simulink model "finalcode"  (R2020a)
settings: Solver=FixedStepDiscrete  StartTime=0.0  StopTime=1  FixedStep=0.0005  RelTol=1e-3  EnableMultiTasking=on
undefined symbols (not defined in the file): acc_calmax1, acc_calmax2, acc_calmin1, acc_calmin2, akemancanshu, angle_middle, bre, bre_calmax, bre_calmin, chasuniujvvvv_hou, chasuniujvvvv_qian, chasuuuu, ecucoder_acal, I_AN01_5K1, I_AN03_5V, I_AN04_5V, kd, kddd, ki, kiii, kp, kppp, leftmax, O_SW06_HS1A, P11111, P22222, PIDmodel, PPPP, rightmax, slip, slip_big, slip_little, slipmodel, T_add, T_del, tiaoshi, TTTTTyouren, vvvv, zhiling
libraries: ec5744lib x305, canmsglib x97, simulink x23
(part 10 of 11)

== matlab function finalcode/Subsystem/run/analog_input/无人意图转译/无人/Subsystem1/进esc控制策略/integral ==
  data: u input; output output; vd input
function output = fcn(u,vd)
    % 赛车PID控制器参数
    kp = 1;
    ki = 0.1;
    kd = 0.1;
    
    % 状态变量
    persistent pre_integral previous_error i
    
    % 初始化状态变量
    if isempty(pre_integral)
        pre_integral = 0;
        previous_error = 0;
        i=0;
    end
        if i>50
            i=0;
        end
    % PID控制器计算
    error = u;
    integral = pre_integral + error*0.02;
    derivative = (error - previous_error)/0.02;
%     integral =0;
    if abs(error)<0.1
        ki=0;
    end
    output = kp * error + ki * integral + kd * derivative;
    
   if vd==0
       output=0;
   end
    % 保存上一个误差用于下次计算
    previous_error = error;
    pre_integral =integral ;
    i=i+1
end

== matlab function finalcode/Subsystem/run/analog_input/无人意图转译/无人/Subsystem1/进esc控制策略/MATLAB Function1 ==
  data: output input; u input; y output; v input; vd input
function y = fcn(output, u,v,vd)
persistent vv
if isempty(vv)
    vv=0;
end
vv=output;
if v-vd>0.1*v
    y=vv;
else
    y=u;
end

== matlab function finalcode/Subsystem/run/analog_input/有人/功率限制jiandan/MATLAB Function ==
  data: u1 input; y output; u2 input; u3 input; u4 input
function y = fcn(u1,u2,u3,u4)
sum=(u1+u2+u3+u4)*594.06/1000/9550;
if sum>75
   a=75/sum;
else
    a=1;
end
y = a;

== matlab function finalcode/Subsystem/run/analog_input/有人/扭矩分配jiandan/MATLAB Function1 ==
  data: fengzhiniuju input; ax input; ay input
function fcn(fengzhiniuju,ax, ay)

end

== matlab function finalcode/Subsystem/run/analog_input/有人/扭矩分配jiandan/MATLAB Function3 ==
  data: M_qian input; M_hou input; youhou output; M input; youqian output; zuohou output; zuoqian output; you input; zuo input
function [youhou,youqian,zuohou,zuoqian] = fcn(M_qian,M_hou,M,you,zuo)
% U=4*u;
r=0.2032;%轮半径
B1=1.18;%左右轮距
B2=1.16;
youqian=you*(M*r/(2*B2)+M_qian);
zuoqian=zuo*(-M*r/(2*B1)+M_qian);
youhou=you*(M*r/(2*B2)+M_hou);
zuohou=zuo*(-M*r/(2*B1)+M_hou);
end

== matlab function finalcode/Subsystem/run/analog_input/无人意图转译/无人/Subsystem1/进esc控制策略/MATLAB Function2 ==
  data: u input; y output
function y = fcn(u)
persistent pre_Torque i
   
    % 初始化状态变量
    if isempty(pre_Torque)
          pre_Torque = 0;
          
        i=0;
    end
    if pre_Torque>u
   Torque= pre_Torque-100;
    else 
     Torque= pre_Torque;   
    end
  
    if  Torque<u
       Torque=u;
    end
    
    pre_Torque = Torque;

    i=i+1;
y = Torque;

== matlab function finalcode/Subsystem/Tx/TX控制器/控制器发送/184左前1/MATLAB Function ==
  data: u input; y output; zhidongesc input; zhidongebs input; huanting input
function y = fcn(u,zhidongesc,zhidongebs,huanting)
 y = u*594.06;
if zhidongesc>1800&&zhidongebs==2
    y = u*594.06;
end
if zhidongesc<1500&&zhidongebs==2
    y=0;
end
if huanting==0
    y=0;
end

== matlab function finalcode/Subsystem/Tx/TX控制器/控制器发送/184左前1/MATLAB Function1 ==
  data: v input; T output; a input
function T = fcn(v,a)
% if a>5
%     y = u;
% elseif a>3&&a<5
%     y=1200;
% else
%     y=800;
% end

if v<6000*1.88e-3
    T=2100;
elseif v>11000*1.88e-3
    T=800;
else
    T=1100;
end

== matlab function finalcode/Subsystem/Tx/TX控制器/控制器发送/184左前1/MATLAB Function3 ==
  data: v input; y output; angle input; vz input; model input
function y = fcn(v, angle, vz,model)
if(angle>3||angle<-3)&&model==3%4650000,4870000,4741002
    y=vz*594.06;
else
    y = v;
end

== matlab function finalcode/Subsystem/Tx/TX控制器/控制器发送/184左前1/MATLAB Function4 ==
  data: NT output; pos input; TargetVelocity input; T output; neg input; wheel_v input; v output
function [NT,T,v]= fcn(pos,TargetVelocity, neg,wheel_v)
persistent new_Torque i
    % 初始化状态变量
    if isempty(new_Torque)
          new_Torque = 0;  
          i=0;
    end
    if neg<0 && i==0;  %反扭
        v=0;
        i=1;
        new_Torque = pos;
    elseif i==1 && neg<0 && new_Torque>neg && new_Torque>=0;
        v=0;
        new_Torque=new_Torque-200;
    elseif i==1 && neg<0 && new_Torque>neg && new_Torque<0;
        v=0;
        new_Torque=new_Torque-50;
    elseif i==1 && neg<0 && new_Torque<=neg;
        v=0;
        new_Torque=neg;
    else %正扭矩情况
        v=TargetVelocity;
        i=0;
    end
    
    if neg<0 && new_Torque>=0
        T=new_Torque;
        NT=0;
    elseif neg<0 && new_Torque<0
        T=0;
        NT=new_Torque;
    else %正扭矩
        T=pos;
        NT=0;
    end
    
    if wheel_v<1
  v=TargetVelocity;
end

== matlab function finalcode/Subsystem/Tx/TX控制器/控制器发送/184左前1/MATLAB Function7 ==
  data: T input; y output; wurenyouya input; youya input; enable input; enable_1 input
function y = fcn(T, wurenyouya,youya, enable, enable_1)
 y = 0;
if wurenyouya>10||youya>500
    y = T;
else
    y=0;
end
if enable==0
    y=0;
end

== matlab function finalcode/Subsystem/Tx/TX控制器/控制器发送/184左前1/复位 ==
  data: enable input; enable_1 input; T input; TargetVelocity output; AMK_TorqueLimitPositive output; enable output; errorreset output; blnverteron output; CAN_dbcon output; v input
function [TargetVelocity,AMK_TorqueLimitPositive,enable,errorreset,blnverteron,CAN_dbcon]= fcn(enable,enable_1,T,v)
if (enable_1==0)
    TargetVelocity=0;
    enable=0;
    errorreset=1;
    blnverteron=0;
    CAN_dbcon=0;
    AMK_TorqueLimitPositive=0;
elseif (enable==0 && enable_1==1)
    TargetVelocity=0;
    enable=1;
    errorreset=0;
    blnverteron=1;
    CAN_dbcon=1;
    AMK_TorqueLimitPositive=0;
elseif (enable==1 && enable_1==1)
    TargetVelocity=v;
    enable=1;
    errorreset=0;
    blnverteron=1;
    CAN_dbcon=1;
    AMK_TorqueLimitPositive=T;
else
    TargetVelocity=0;
    enable=0;
    errorreset=1;
    blnverteron=0;
    CAN_dbcon=0;
    AMK_TorqueLimitPositive=0;
end

end

== matlab function finalcode/Subsystem/Tx/TX控制器/速度/185右前/MATLAB Function4 ==
  data: u input; y output; zhidongesc input; zhidongebs input; huanting input
function y = fcn(u,zhidongesc,zhidongebs,huanting)
 y = u*594.06;
if zhidongesc>1800&&zhidongebs==2
    y = u*594.06;
end
if zhidongesc<1500&&zhidongebs==2
    y=0;
end
if huanting~=0
    y=0;
end

== matlab function finalcode/Subsystem/Tx/TX控制器/控制器发送/184左前1/无人模式速度判断 ==
  data: u input; y output; zhidongesc input; zhidongebs input; huanting input
function y = fcn(u,zhidongesc,zhidongebs,huanting)
 y = u*594.06;
if zhidongesc>1800&&zhidongebs==2
    y = u*594.06;
end
if zhidongesc<1500&&zhidongebs==2
    y=0;
end
if huanting~=0
    y=0;
end

== matlab function finalcode/Subsystem/Tx/TX控制器/控制器发送/184左前1/有人无人扭矩转换 ==
  data: angle input; baziniujv input; v input; youren input; T output; model input
function T = fcn(angle, baziniujv, v,youren, model)
% if a>5
%     y = u;
% elseif a>3&&a<5
%     y=1200;
% else
%     y=800;
% end

if model==0||model==9||model==10   %有人模式，调试模式
    T=youren;
elseif model==3||abs(angle)>3  %wurenbazi
        if baziniujv==0
            T_bazi=2100;
        else
            T_bazi=baziniujv;
        end
        
    if v<10000*1.88e-3
        T=T_bazi;
    elseif v>11000*1.88e-3
        T=800;
    else
        T=1100;
   end
else                    %无人模式
   if v<6000*1.88e-3
     T=2100;
    elseif v>11000*1.88e-3
        T=800;
    else
        T=1100;
   end
end

== matlab function finalcode/Subsystem/Tx/TX控制器/控制器发送/184左前1/有人无人速度转换 ==
  data: v input; y output; angle input; vz input; model input; zhidong input; T input; vk input; v_youren input
function y = fcn(v, angle, vz,model, zhidong, T, vk, v_youren)
if model==0||model==9||model==10  %有人模式/无人检查（电气）
    if zhidong==0
       y=v_youren;
    else 
        y=0;
    end
else                    %无人模式
    if model==3 %4650000,4870000,4741002 大角度且八字
        y=vz*594.06;
    elseif T >10
        y=0;
        if vk<1
            y=v*594.06;
        end
    else
        y = v;  
    end    
end

== matlab function finalcode/Subsystem/Tx/TX控制器/控制器发送/184左前1/能量回收功率限制/MATLAB Function ==
  data: youya input; T output; model input; status input; wurenyouya input; Negativ_T input
function T = fcn(youya, model, status, wurenyouya, Negativ_T)
    if model == 0||model==10  %有人模式
        if youya>500
            T = (youya-500)*Negativ_T/4000;%最大反扭1000
            if youya>4500
                T = Negativ_T;
            end
        else
            T = 0;
        end
        
    elseif model~=0&&model~=9&&model~=2  %无人模式
        if wurenyouya>10
            T = -wurenyouya
        elseif status==5||status==7
                T=-1500; 
           % T = -(wurenyouya-500)/4;%最大反扭1000
            %if wurenyouya>500&&status==5
             %   T = -1000;
            %end
        else
            T = 0;
        end
    else
        T = 0;
end

== matlab function finalcode/Subsystem/Tx/TX控制器/控制器发送/184左前1/能量回收功率限制/MATLAB Function1 ==
  data: er_T input; T output; Iq input; L_Iq input; L_er_T input
function T = fcn(er_T, Iq, L_Iq,L_er_T)
if er_T<0
    if abs(Iq)>abs(L_Iq)
        T = -abs(L_er_T);

    else
        T = -abs(er_T);
    end
else
    T=0;
end

== matlab function finalcode/Subsystem/Tx/TX控制器/控制器发送/185右前1/MATLAB Function ==
  data: u input; y output; zhidongesc input; zhidongebs input
function y = fcn(u,zhidongesc,zhidongebs)
 y = u*594.06;
if zhidongesc>1800&&zhidongebs==2
    y = u*594.06;
end
if zhidongesc<1500&&zhidongebs==2
    y=0;
end

== matlab function finalcode/Subsystem/Tx/TX控制器/控制器发送/185右前1/MATLAB Function1 ==
  data: v input; T output; a input
function T = fcn(v,a)
% if a>5
%     y = u;
% elseif a>3&&a<5
%     y=1200;
% else
%     y=800;
% end

if v<6000*1.88e-3
    T=2100;
elseif v>11000*1.88e-3
    T=800;
else
    T=1100;
end

== matlab function finalcode/Subsystem/Tx/TX控制器/控制器发送/185右前1/MATLAB Function2 ==
  data: enable input; enable_1 input; T input; TargetVelocity output; AMK_TorqueLimitPositive output; enable output; errorreset output; blnverteron output; CAN_dbcon output; v input
function [TargetVelocity,AMK_TorqueLimitPositive,enable,errorreset,blnverteron,CAN_dbcon]= fcn(enable,enable_1,T,v)
if (enable_1==0)
    TargetVelocity=0;
    enable=0;
    errorreset=1;
    blnverteron=0;
    CAN_dbcon=0;
    AMK_TorqueLimitPositive=0;
elseif (enable==0 && enable_1==1)
    TargetVelocity=0;
    enable=1;
    errorreset=0;
    blnverteron=1;
    CAN_dbcon=1;
    AMK_TorqueLimitPositive=0;
elseif (enable==1 && enable_1==1)
    TargetVelocity=v;
    enable=1;
    errorreset=0;
    blnverteron=1;
    CAN_dbcon=1;
    AMK_TorqueLimitPositive=T;
else
    TargetVelocity=0;
    enable=0;
    errorreset=1;
    blnverteron=0;
    CAN_dbcon=0;
    AMK_TorqueLimitPositive=0;
end

end

== matlab function finalcode/Subsystem/Tx/TX控制器/速度/185右前/MATLAB Function5 ==
  data: v input; y output; angle input; vz input; model input
function y = fcn(v, angle, vz,model)
if(angle>3||angle<-3)&&model==3%4650000,4870000,4741002
    y=vz*594.06;
else
    y = v;
end

== matlab function finalcode/Subsystem/Tx/TX控制器/控制器发送/185右前1/MATLAB Function3 ==
  data: v input; y output; angle input; vz input; model input
function y = fcn(v, angle, vz,model)
if (angle>3||angle<-3)&&model==3%4650000,4870000,4741002
    y=vz*594.06;
else
    y = v;
end

== matlab function finalcode/Subsystem/Tx/TX控制器/控制器发送/185右前1/MATLAB Function4 ==
  data: u input; y output; zhidongesc input; zhidongebs input; huanting input
function y = fcn(u,zhidongesc,zhidongebs,huanting)
 y = u*594.06;
if zhidongesc>1800&&zhidongebs==2
    y = u*594.06;
end
if zhidongesc<1500&&zhidongebs==2
    y=0;
end
if huanting~=0
    y=0;
end

== matlab function finalcode/Subsystem/Tx/TX控制器/控制器发送/185右前1/vvv ==
  data: v input; y output; angle input; vz input; model input; zhidong input; T input; vk input; v_youren input
function y = fcn(v, angle, vz,model, zhidong, T, vk, v_youren)
if model==0||model==9||model==10  %有人模式/无人检查（电气）
    if zhidong==0
       y=v_youren;
    else 
        y=0;
    end
else                    %无人模式
    if model==3 %4650000,4870000,4741002 大角度和八字状态
        y=vz*594.06;
    elseif T >10
        y=0;
        if vk<1
            y=v*594.06;
        end
    else
        y = v;
    end   
end

== matlab function finalcode/Subsystem/Tx/TX控制器/控制器发送/185右前1/MATLAB Function6 ==
  data: angle input; baziniujv input; v input; youren input; T output; model input
function T = fcn(angle, baziniujv, v,youren, model)
% if a>5
%     y = u;
% elseif a>3&&a<5
%     y=1200;
% else
%     y=800;
% end

if model==0||model==9||model==10   %有人模式，调试模式
    T=youren;
elseif model==3||abs(angle)>3  %wurenbazi
        if baziniujv==0
            T_bazi=2100;
        else
            T_bazi=baziniujv;
        end
        
    if v<10000*1.88e-3
        T=T_bazi;
    elseif v>11000*1.88e-3
        T=800;
    else
        T=1100;
   end
else                    %无人模式
   if v<6000*1.88e-3
     T=2100;
    elseif v>11000*1.88e-3
        T=800;
    else
        T=1100;
   end
end

== matlab function finalcode/Subsystem/Tx/TX控制器/控制器发送/185右前1/MATLAB Function7 ==
  data: T input; y output; wurenyouya input; youya input; enable input; enable_1 input
function y = fcn(T, wurenyouya,youya, enable, enable_1)
 y = 0;
if wurenyouya>10||youya>500
    y = T;
else
    y=0;
end
if enable==0
    y=0;
end

== matlab function finalcode/Subsystem/Tx/TX控制器/控制器发送/185右前1/MATLAB Function8 ==
  data: pos input; TargetVelocity input; NT output; T output; neg input; wheel_v input; v output
function [NT,T,v]= fcn(pos,TargetVelocity, neg,wheel_v)
persistent new_Torque i
    % 初始化状态变量
    if isempty(new_Torque)
          new_Torque = 0;  
          i=0;
    end
    if neg<0 && i==0;  %反扭
        v=0;
        i=1;
        new_Torque = pos;
    elseif i==1 && neg<0 && new_Torque>neg && new_Torque>=0;
        v=0;
        new_Torque=new_Torque-200;
    elseif i==1 && neg<0 && new_Torque>neg && new_Torque<0;
        v=0;
        new_Torque=new_Torque-50;
    elseif i==1 && neg<0 && new_Torque<=neg;
        v=0;
        new_Torque=neg;
    else %正扭矩情况
        v=TargetVelocity;
        i=0;
    end
    
    if neg<0 && new_Torque>=0
        T=new_Torque;
        NT=0;
    elseif neg<0 && new_Torque<0
        T=0;
        NT=new_Torque;
    else %正扭矩
        T=pos;
        NT=0;
    end
    
    if wheel_v<1
  v=TargetVelocity;
end

== matlab function finalcode/Subsystem/Tx/TX控制器/控制器发送/185右前1/能量回收功率限制/MATLAB Function ==
  data: youya input; T output; model input; status input; wurenyouya input; Negativ_T input
function T = fcn(youya, model, status, wurenyouya, Negativ_T)
    if model == 0||model==10  %有人模式
        if youya>500
            T = (youya-500)*Negativ_T/4000;%最大反扭1000
            if youya>4500
                T = Negativ_T;
            end
        else
            T = 0;
        end
        
    elseif model~=0&&model~=9&&model~=2  %无人模式
        if wurenyouya>10
            T = -wurenyouya
        elseif status==5||status==7
                T=-1500;
           % T = -(wurenyouya-500)/4;%最大反扭1000
            %if wurenyouya>500&&status==5
             %   T = -1000;
            %end
        else
            T = 0;
        end
    else
        T = 0;
end

== matlab function finalcode/Subsystem/Tx/TX控制器/控制器发送/185右前1/能量回收功率限制/MATLAB Function1 ==
  data: er_T input; T output; Iq input; L_Iq input; L_er_T input
function T = fcn(er_T, Iq, L_Iq,L_er_T)
if er_T<0
    if abs(Iq)>abs(L_Iq)
        T = -abs(L_er_T);

    else
        T = -abs(er_T);
    end
else
    T=0;
end

== matlab function finalcode/Subsystem/Tx/TX控制器/控制器发送/188右后1/MATLAB Function ==
  data: u input; y output; zhidongesc input; zhidongebs input
function y = fcn(u,zhidongesc,zhidongebs)
 y = u*594.06;
if zhidongesc>1800&&zhidongebs==2
    y = u*594.06;
end
if zhidongesc<1500&&zhidongebs==2
    y=0;
end

== matlab function finalcode/Subsystem/Tx/TX控制器/控制器发送/188右后1/MATLAB Function1 ==
  data: v input; T output; a input
function T = fcn(v,a)
% if a>5
%     y = u;
% elseif a>3&&a<5
%     y=1200;
% else
%     y=800;
% end

if v<6000*1.88e-3
    T=2100;
elseif v>11000*1.88e-3
    T=800;
else
    T=1100;
end

== matlab function finalcode/Subsystem/Tx/TX控制器/速度/185右前/MATLAB Function6 ==
  data: v input; T output; a input
function T = fcn(v,a)
% if a>5
%     y = u;
% elseif a>3&&a<5
%     y=1200;
% else
%     y=800;
% end

if v<6000*1.88e-3
    T=2100;
elseif v>11000*1.88e-3
    T=800;
else
    T=1100;
end

== matlab function finalcode/Subsystem/Tx/TX控制器/控制器发送/188右后1/MATLAB Function2 ==
  data: enable input; enable_1 input; T input; TargetVelocity output; AMK_TorqueLimitPositive output; enable output; errorreset output; blnverteron output; CAN_dbcon output; v input
function [TargetVelocity,AMK_TorqueLimitPositive,enable,errorreset,blnverteron,CAN_dbcon]= fcn(enable,enable_1,T,v)
if (enable_1==0)
    TargetVelocity=0;
    enable=0;
    errorreset=1;
    blnverteron=0;
    CAN_dbcon=0;
    AMK_TorqueLimitPositive=0;
elseif (enable==0 && enable_1==1)
    TargetVelocity=0;
    enable=1;
    errorreset=0;
    blnverteron=1;
    CAN_dbcon=1;
    AMK_TorqueLimitPositive=0;
elseif (enable==1 && enable_1==1)
    TargetVelocity=v;
    enable=1;
    errorreset=0;
    blnverteron=1;
    CAN_dbcon=1;
    AMK_TorqueLimitPositive=T;
else
    TargetVelocity=0;
    enable=0;
    errorreset=1;
    blnverteron=0;
    CAN_dbcon=0;
    AMK_TorqueLimitPositive=0;
end

end

== matlab function finalcode/Subsystem/Tx/TX控制器/控制器发送/188右后1/MATLAB Function3 ==
  data: v input; y output; angle input; vz input; model input
function y = fcn(v, angle,vz,model)
if (angle>3||angle<-3)&&model==3%4650000,4870000,4741002
    y=vz*594.06;
else
    y = v;
end

== matlab function finalcode/Subsystem/Tx/TX控制器/控制器发送/188右后1/MATLAB Function4 ==
  data: u input; y output; zhidongesc input; zhidongebs input; huanting input
function y = fcn(u,zhidongesc,zhidongebs,huanting)
 y = u*594.06;
if zhidongesc>1800&&zhidongebs==2
    y = u*594.06;
end
if zhidongesc<1500&&zhidongebs==2
    y=0;
end
if huanting~=0
    y=0;
end

== matlab function finalcode/Subsystem/Tx/TX控制器/控制器发送/188右后1/MATLAB Function5 ==
  data: v input; y output; angle input; vz input; model input; zhidong input; T input; vk input; v_youren input
function y = fcn(v, angle, vz,model, zhidong, T, vk, v_youren)
if model==0||model==9||model==10  %有人模式/无人检查（电气）
    if zhidong==0
       y=v_youren;
    else 
        y=0;
    end
else                    %无人模式
    if model==3 %4650000,4870000,4741002 大角度和八字状态
        y=vz*594.06;
    elseif T >10
        y=0;
        if vk<1
            y=v*594.06;
        end
    else
        y = v;
    end    
end

== matlab function finalcode/Subsystem/Tx/TX控制器/控制器发送/188右后1/MATLAB Function6 ==
  data: T input; y output; wurenyouya input; youya input; enable input; enable_1 input
function y = fcn(T, wurenyouya,youya, enable, enable_1)
 y = 0;
if wurenyouya>10||youya>500
    y = T;
else
    y=0;
end
if enable==0
    y=0;
end

== matlab function finalcode/Subsystem/Tx/TX控制器/控制器发送/188右后1/MATLAB Function7 ==
  data: angle input; baziniujv input; v input; youren input; T output; model input
function T = fcn(angle, baziniujv, v,youren, model)
% if a>5
%     y = u;
% elseif a>3&&a<5
%     y=1200;
% else
%     y=800;
% end

if model==0||model==9||model==10   %有人模式，调试模式
    T=youren;
elseif model==3||abs(angle)>3  %wurenbazi
        if baziniujv==0
            T_bazi=2100;
        else
            T_bazi=baziniujv;
        end
        
    if v<10000*1.88e-3
        T=T_bazi;
    elseif v>11000*1.88e-3
        T=800;
    else
        T=1100;
   end
else                    %无人模式
   if v<6000*1.88e-3
     T=2100;
    elseif v>11000*1.88e-3
        T=800;
    else
        T=1100;
   end
end

== matlab function finalcode/Subsystem/Tx/TX控制器/控制器发送/188右后1/MATLAB Function9 ==
  data: pos input; TargetVelocity input; NT output; T output; neg input; wheel_v input; v output
function [NT,T,v]= fcn(pos,TargetVelocity, neg,wheel_v)
persistent new_Torque i
    % 初始化状态变量
    if isempty(new_Torque)
          new_Torque = 0;  
          i=0;
    end
    if neg<0 && i==0;  %反扭
        v=0;
        i=1;
        new_Torque = pos;
    elseif i==1 && neg<0 && new_Torque>neg && new_Torque>=0;
        v=0;
        new_Torque=new_Torque-200;
    elseif i==1 && neg<0 && new_Torque>neg && new_Torque<0;
        v=0;
        new_Torque=new_Torque-50;
    elseif i==1 && neg<0 && new_Torque<=neg;
        v=0;
        new_Torque=neg;
    else %正扭矩情况
        v=TargetVelocity;
        i=0;
    end
    
    if neg<0 && new_Torque>=0
        T=new_Torque;
        NT=0;
    elseif neg<0 && new_Torque<0
        T=0;
        NT=new_Torque;
    else %正扭矩
        T=pos;
        NT=0;
    end
    
    if wheel_v<1
  v=TargetVelocity;
end

== matlab function finalcode/Subsystem/Tx/Toworkstation/toworkstation/toworkstation/MATLAB Function ==
  data: T input; y output; NT input
function y = fcn(T, NT)

y = T;
if NT<-10
    y=NT;
end

== matlab function finalcode/Subsystem/Tx/TX控制器/控制器发送/188右后1/能量回收功率限制/MATLAB Function ==
  data: youya input; T output; model input; status input; wurenyouya input; Negativ_T input
function T = fcn(youya, model, status, wurenyouya, Negativ_T)
    if model == 0||model==10  %有人模式
        if youya>500
            T = (youya-500)*Negativ_T/4000;%最大反扭1000
            if youya>4500
                T = Negativ_T;
            end
        else
            T = 0;
        end
        
    elseif model~=0&&model~=9&&model~=2  %无人模式
        if wurenyouya>10
            T = -wurenyouya
        elseif status==5||status==7
                T=-1500;
           % T = -(wurenyouya-500)/4;%最大反扭1000
            %if wurenyouya>500&&status==5
             %   T = -1000;
            %end
        else
            T = 0;
        end
    else
        T = 0;
end

== matlab function finalcode/Subsystem/Tx/TX控制器/控制器发送/188右后1/能量回收功率限制/MATLAB Function1 ==
  data: er_T input; T output; Iq input; L_Iq input; L_er_T input
function T = fcn(er_T, Iq, L_Iq,L_er_T)
if er_T<0
    if abs(Iq)>abs(L_Iq)
        T = -abs(L_er_T);

    else
        T = -abs(er_T);
    end
else
    T=0;
end

== matlab function finalcode/Subsystem/Tx/TX控制器/控制器发送/189左后1/MATLAB Function ==
  data: u input; y output; zhidongesc input; zhidongebs input
function y = fcn(u,zhidongesc,zhidongebs)
 y = u*594.06;
if zhidongesc>1800&&zhidongebs==2
    y = u*594.06;
end
if zhidongesc<1500&&zhidongebs==2
    y=0;
end

== matlab function finalcode/Subsystem/Tx/TX控制器/控制器发送/189左后1/MATLAB Function1 ==
  data: v input; T output; a input
function T = fcn(v,a)
% if a>5
%     y = u;
% elseif a>3&&a<5
%     y=1200;
% else
%     y=800;
% end

if v<6000*1.88e-3
    T=2100;
elseif v>11000*1.88e-3
    T=800;
else
    T=1100;
end

== matlab function finalcode/Subsystem/Tx/TX控制器/控制器发送/189左后1/MATLAB Function2 ==
  data: enable input; enable_1 input; T input; TargetVelocity output; AMK_TorqueLimitPositive output; enable output; errorreset output; blnverteron output; CAN_dbcon output; v input
function [TargetVelocity,AMK_TorqueLimitPositive,enable,errorreset,blnverteron,CAN_dbcon]= fcn(enable,enable_1,T,v)
if (enable_1==0)
    TargetVelocity=0;
    enable=0;
    errorreset=1;
    blnverteron=0;
    CAN_dbcon=0;
    AMK_TorqueLimitPositive=0;
elseif (enable==0 && enable_1==1)
    TargetVelocity=0;
    enable=1;
    errorreset=0;
    blnverteron=1;
    CAN_dbcon=1;
    AMK_TorqueLimitPositive=0;
elseif (enable==1 && enable_1==1)
    TargetVelocity=v;
    enable=1;
    errorreset=0;
    blnverteron=1;
    CAN_dbcon=1;
    AMK_TorqueLimitPositive=T;
else
    TargetVelocity=0;
    enable=0;
    errorreset=1;
    blnverteron=0;
    CAN_dbcon=0;
    AMK_TorqueLimitPositive=0;
end

end

== matlab function finalcode/Subsystem/Tx/TX控制器/控制器发送/189左后1/MATLAB Function3 ==
  data: v input; y output; angle input; vz input; model input
function y = fcn(v, angle, vz,model)
if (angle>3||angle<-3)&&model==3%4650000,4870000,4741002
    y=vz*594.06;
else
    y = v;
end

== matlab function finalcode/Subsystem/Tx/TX控制器/控制器发送/189左后1/MATLAB Function4 ==
  data: u input; y output; zhidongesc input; zhidongebs input; huanting input
function y = fcn(u,zhidongesc,zhidongebs,huanting)
 y = u*594.06;
if zhidongesc>1800&&zhidongebs==2
    y = u*594.06;
end
if zhidongesc<1500&&zhidongebs==2
    y=0;
end
if huanting~=0
    y=0;
end

== matlab function finalcode/Subsystem/Tx/Toworkstation/toworkstation/toworkstation/MATLAB Function1 ==
  data: T input; y output; NT input
function y = fcn(T, NT)

y = T;
if NT<-10
    y=NT;
end

== matlab function finalcode/Subsystem/Tx/TX控制器/控制器发送/189左后1/MATLAB Function5 ==
  data: v input; y output; angle input; vz input; model input; zhidong input; T input; vk input; v_youren input
function y = fcn(v, angle, vz,model, zhidong, T, vk, v_youren)
if model==0||model==9||model==10  %有人模式/无人检查（电气）
    if zhidong==0
       y=v_youren;
    else 
        y=0;
    end
else                    %无人模式
    if model==3 %4650000,4870000,4741002 大角度和八字状态
        y=vz*594.06;
    elseif T >10
        y=0;
        if vk<1
            y=v*594.06;
        end
    else
        y = v;   
    end     
end

== matlab function finalcode/Subsystem/Tx/TX控制器/控制器发送/189左后1/MATLAB Function6 ==
  data: angle input; baziniujv input; v input; youren input; T output; model input
function T = fcn(angle, baziniujv, v,youren, model)
% if a>5
%     y = u;
% elseif a>3&&a<5
%     y=1200;
% else
%     y=800;
% end

if model==0||model==9||model==10   %有人模式，调试模式
    T=youren;
elseif model==3||abs(angle)>3  %wurenbazi
        if baziniujv==0
            T_bazi=2100;
        else
            T_bazi=baziniujv;
        end
        
    if v<10000*1.88e-3
        T=T_bazi;
    elseif v>11000*1.88e-3
        T=800;
    else
        T=1100;
   end
else                    %无人模式
   if v<6000*1.88e-3
     T=2100;
    elseif v>11000*1.88e-3
        T=800;
    else
        T=1100;
   end
end

== matlab function finalcode/Subsystem/Tx/TX控制器/控制器发送/189左后1/MATLAB Function7 ==
  data: T input; y output; wurenyouya input; youya input; enable input; enable_1 input
function y = fcn(T, wurenyouya,youya, enable, enable_1)
 y = 0;
if wurenyouya>10||youya>500
    y = T;
else
    y=0;
end
if enable==0
    y=0;
end

== matlab function finalcode/Subsystem/Tx/TX控制器/控制器发送/189左后1/MATLAB Function9 ==
  data: pos input; TargetVelocity input; NT output; T output; neg input; v output; wheel_v input
function [NT,T,v]= fcn(pos,TargetVelocity, neg,wheel_v)
persistent new_Torque i
    % 初始化状态变量
    if isempty(new_Torque)
          new_Torque = 0;  
          i=0;
    end
    if neg<0 && i==0;  %反扭
        v=0;
        i=1;
        new_Torque = pos;
    elseif i==1 && neg<0 && new_Torque>neg && new_Torque>=0;
        v=0;
        new_Torque=new_Torque-200;
    elseif i==1 && neg<0 && new_Torque>neg && new_Torque<0;
        v=0;
        new_Torque=new_Torque-50;
    elseif i==1 && neg<0 && new_Torque<=neg;
        v=0;
        new_Torque=neg;
    else %正扭矩情况
        v=TargetVelocity;
        i=0;
    end
    
    if neg<0 && new_Torque>=0
        T=new_Torque;
        NT=0;
    elseif neg<0 && new_Torque<0
        T=0;
        NT=new_Torque;
    else %正扭矩
        T=pos;
        NT=0;
    end
    
    if wheel_v<1
  v=TargetVelocity;
end

== matlab function finalcode/Subsystem/Tx/TX控制器/控制器发送/189左后1/能量回收功率限制/MATLAB Function ==
  data: youya input; T output; model input; status input; wurenyouya input; Negativ_T input
function T = fcn(youya, model, status, wurenyouya, Negativ_T)
    if model == 0||model==10  %有人模式
        if youya>500
            T = (youya-500)*Negativ_T/4000;%最大反扭1000
            if youya>4500
                T = Negativ_T;
            end
        else
            T = 0;
        end
        
    elseif model~=0&&model~=9&&model~=2  %无人模式
        if wurenyouya>10
            T = -wurenyouya
        elseif status==5||status==7
                T=-1500;
           % T = -(wurenyouya-500)/4;%最大反扭1000
            %if wurenyouya>500&&status==5
             %   T = -1000;
            %end
        else
            T = 0;
        end
    else
        T = 0;
end

== matlab function finalcode/Subsystem/Tx/TX控制器/控制器发送/189左后1/能量回收功率限制/MATLAB Function1 ==
  data: er_T input; T output; Iq input; L_Iq input; L_er_T input
function T = fcn(er_T, Iq, L_Iq,L_er_T)
if er_T<0
    if abs(Iq)>abs(L_Iq)
        T = -abs(L_er_T);

    else
        T = -abs(er_T);
    end
else
    T=0;
end

== matlab function finalcode/Subsystem/Tx/Toworkstation/toworkstation/toworkstation/MATLAB Function2 ==
  data: T input; y output; NT input
function y = fcn(T, NT)

y = T;
if NT<-10
    y=NT;
end

== matlab function finalcode/Subsystem/Tx/Toworkstation/toworkstation/toworkstation/MATLAB Function3 ==
  data: T input; y output; NT input
function y = fcn(T, NT)

y = T;
if NT<-10
    y=NT;
end

== matlab function finalcode/Subsystem/Rx/工作站/Subsystem3/Subsystem/MATLAB Function5 ==
  data: steer input; u input; y output; CANOK_20 input
function y = fcn(steer, u, CANOK_20)

% 初始化位数计数
num_digits = 0; 
% 处理0的情况
if u == 0
    num_digits = 1;
else
    % 计算位数
    num = abs(u);
    while num > 0
        num = floor(num / 10);
        num_digits = num_digits + 1;
    end
end
    divisor = 10 ^ num_digits;
    decimal = u / divisor;
    
    if steer>=0
        y=decimal;
    else
        y=-decimal;
    end
 
%     if CANOK_20==0
%     y=0;
%     end
end

== matlab function finalcode/Subsystem/Rx/工作站/Subsystem3/Subsystem/MATLAB Function3 ==
  data: steer input; u input; y output; CANOK_20 input
function y = fcn(steer, u,CANOK_20)
        y=u/100;

== matlab function finalcode/无人TX/Toworkstation/MATLAB Function ==
  data: u input; y output
function y = fcn(u)
if u~=0&&u~=9&&u~=2
    y=1;
else
    y=0;
end

== matlab function finalcode/Subsystem/Tx/TX控制器/速度/184左前/MATLAB Function2 ==
  data: enable input; enable_1 input; T input; TargetVelocity output; AMK_TorqueLimitPositive output; enable output; errorreset output; blnverteron output; CAN_dbcon output; v input
function [TargetVelocity,AMK_TorqueLimitPositive,enable,errorreset,blnverteron,CAN_dbcon]= fcn(enable,enable_1,T,v)
if (enable_1==0)
    TargetVelocity=0;
    enable=0;
    errorreset=1;
    blnverteron=0;
    CAN_dbcon=0;
    AMK_TorqueLimitPositive=0;
elseif (enable==0 && enable_1==1)
    TargetVelocity=2000;
    enable=1;
    errorreset=0;
    blnverteron=1;
    CAN_dbcon=1;
    AMK_TorqueLimitPositive=0;
elseif (enable==1 && enable_1==1)
    TargetVelocity=2000;
    enable=1;
    errorreset=0;
    blnverteron=1;
    CAN_dbcon=1;
    AMK_TorqueLimitPositive=T;
else
    TargetVelocity=0;
    enable=0;
    errorreset=1;
    blnverteron=0;
    CAN_dbcon=0;
    AMK_TorqueLimitPositive=0;
end

end

== matlab function finalcode/无人TX/Toworkstation/toworkstation/toworkstation/MATLAB Function ==
  data: T input; y output; NT input
function y = fcn(T, NT)

y = T;
if NT<-10
    y=NT;
end

== matlab function finalcode/无人TX/Toworkstation/toworkstation/toworkstation/MATLAB Function1 ==
  data: T input; y output; NT input
function y = fcn(T, NT)

y = T;
if NT<-10
    y=NT;
end

== matlab function finalcode/无人TX/Toworkstation/toworkstation/toworkstation/MATLAB Function2 ==
  data: T input; y output; NT input
function y = fcn(T, NT)

y = T;
if NT<-10
    y=NT;
end

== matlab function finalcode/Subsystem/Rx/lcu——receive/Subsystem1/Subsystem/MATLAB Function ==
  data: m input; y1 output; y2 output; y3 output
function [y1,y2,y3] = fcn(m)
V=zeros(1,3);
a=2;i=3;
while i>0
    V(1,i)=mod(m,a);
    m=fix(m/2);
    i=i-1;
end  
y1 = V(1,3);
y2=V(1,2);
y3=V(1,1);
end

== matlab function finalcode/Subsystem/Rx/lcu——receive/Subsystem1/Subsystem/MATLAB Function1 ==
  data: u input; y output
function y = fcn(u)
if u==7
    y = 1;
else
    y=0;
end
end

== matlab function finalcode/无人TX/Toworkstation/toworkstation/toworkstation/MATLAB Function3 ==
  data: T input; y output; NT input
function y = fcn(T, NT)

y = T;
if NT<-10
    y=NT;
end

== matlab function finalcode/Subsystem/Rx/工作站/Subsystem3/Subsystem/MATLAB Function6 ==
  data: u input; y output; CANOK_20 input
function y = fcn(u, CANOK_20)


% 初始化位数计数
num_digits = 0; 
% 处理0的情况
if u == 0
    num_digits = 1;
else
    % 计算位数
    num = abs(u);
    while num > 0
        num = floor(num / 10);
        num_digits = num_digits + 1;
    end
end
    divisor = 10 ^ num_digits;
    decimal = u / divisor;
    if u>0
        y=decimal;
    else
        y=-decimal;
    end
    if CANOK_20==0
    y=0;
    end
end

== matlab function finalcode/Subsystem/Rx/工作站/Subsystem3/Subsystem/MATLAB Function7 ==
  data: u input; y output; CANOK_20 input
function y = fcn(u,CANOK_20)
if CANOK_20==0
    y=0;
else
    y=u;
end

== matlab function finalcode/Subsystem/Rx/工作站/Subsystem3/Subsystem/MATLAB Function8 ==
  data: u input; y output; CANOK_20 input
function y = fcn(u, CANOK_20)
    if u==0
        y=0;
    else
        y=u/100;
    end
    
    if CANOK_20==0
    y=0;
    end
end

== matlab function finalcode/Subsystem/run/analog_input/无人意图转译/无人/Subsystem1/进esc控制策略/MATLAB Function3 ==
  data: v input; y output; v_k input
function y = fcn( v, v_k)
persistent pre_Torque a
   
    % 初始化状态变量
    if isempty(pre_Torque)
          pre_Torque = 0; 
            a=0;
    end
if v_k>v
    a=v-v_k;
else
    a=0;
end

if a<-0.5
    y=a;
else
    y=0;
end

== matlab function finalcode/Subsystem/Tx/TX控制器/控制器发送/184左前1/能量回收功率限制/P功率 ==
  data: P input; P1 input; P2 input; model input; y output
function y = fcn(P, P1, P2, model)
y=P;
if model==4||model==5  %循迹模式
    y=P1;
elseif model==1
    y=P2;
end

== matlab function finalcode/Subsystem/Tx/TX控制器/控制器发送/185右前1/能量回收功率限制/MATLAB Function2 ==
  data: P input; P1 input; P2 input; model input; y output
function y = fcn(P, P1, P2, model)
y=P;
if model==4||model==5  %循迹模式
    y=P1;
elseif model==1
    y=P2;
end

== matlab function finalcode/Subsystem/Tx/TX控制器/控制器发送/189左后1/能量回收功率限制/MATLAB Function2 ==
  data: P input; P1 input; P2 input; model input; y output
function y = fcn(P, P1, P2, model)
y=P;
if model==4||model==5  %循迹模式
    y=P1;
elseif model==1
    y=P2;
end

== matlab function finalcode/Subsystem/Tx/TX控制器/控制器发送/188右后1/能量回收功率限制/MATLAB Function2 ==
  data: P input; P1 input; P2 input; model input; y output
function y = fcn(P, P1, P2, model)
y=P;
if model==4||model==5  %循迹模式
    y=P1;
elseif model==1
    y=P2;
end

== matlab function finalcode/Subsystem/Tx/MATLAB Function ==
  data: u input; y output
function y = fcn(u)
if u==8
    y=1;
else
    y=0;
end

== matlab function finalcode/Subsystem/Tx/TX控制器/控制器发送/184左前1/滑移率控制 ==
  data: model input; v_e input; v_w input; v input; slipp input; y output; slip_little input; slip_big input
function y = fcn(model, v_e, v_w, v, slipp, slip_little, slip_big)
    persistent i j
    if isempty(i)
        i=1;
        j=1;
    end
if model==0
    y=v_e;
else
    slip=(v-v_w)/v;
    y=v_e;

    if abs(v_e-v_w)>0.5
        if slip_little==0  %调试用
            slip1=0.8;
        else
            slip1=slip_little;
        end
        if slip_big==0
            slip2=1.25;
        else
            slip2=slip_big;
        end
        if slipp==0
            slippp=0.21;
        else
            slippp=slipp;
        end
    if slip>slippp&&v_w>3; %减速，加大轮速
        y=j*v;
        i=i+1;
        j=0.99^i;
        if j<slip1
            j=slip1;
        end
    elseif slip<-slippp&&v_w>2%加速，缓加速
        y=j*v;
        i=i+1;
        j=1.01^i;
        if j>slip2
            j=slip2;
        end
    else
        y=v_e;
        i=1;
    end
    
    else
        y=v_e;
    end
    
    if v_e==0;
        y=0;
    end
end

== matlab function finalcode/Subsystem/run/analog_input/无人意图转译/无人/Subsystem1/MATLAB Function1 ==
  data: v input; model input; a1 input; a2 input; a3 input; a4 input; v1 input; v2 input; v3 input; v4 input; y1 output; y2 output; y3 output; y4 output
function [y1,y2,y3,y4] = fcn(v, model, a1, a2, a3, a4,v1,v2,v3,v4)
if model==3&&v>3
    u1=0;
    u2=0;
    u3=0;
    u4=0;
    if a1>0.5
        u1=a1*247/4;
    elseif a2>0.5
        u2=a2*247/4;
    elseif a3>0.5
        u3=a3*247/4;
    elseif a4>0.5
        u4=a4*247/4;
    end
    y1=u1;
    y2=u2;
    y3=u3;
    y4=u4;
else 
    y1=v1;
    y2=v2;
    y3=v3;
    y4=v4;
end

== matlab function finalcode/Subsystem/Tx/TX控制器/速度/184左前/MATLAB Function4 ==
  data: u input; y output; zhidongesc input; zhidongebs input; huanting input
function y = fcn(u,zhidongesc,zhidongebs,huanting)
 y = u*594.06;
if zhidongesc>1800&&zhidongebs==2
    y = u*594.06;
end
if zhidongesc<1500&&zhidongebs==2
    y=0;
end
if huanting~=0
    y=0;
end

== matlab function finalcode/Subsystem/Tx/TX控制器/控制器发送/185右前1/MATLAB Function9 ==
  data: model input; v_e input; v_w input; v input; y output; slipp input; slip_little input; slip_big input
function y = fcn(model, v_e, v_w, v, slipp, slip_little, slip_big)
    persistent i j
    if isempty(i)
        i=1;
        j=1;
    end
if model==0
    y=v_e;
else
    slip=(v-v_w)/v;
    y=v_e;

    if abs(v_e-v_w)>0.5
        if slip_little==0  %调试用
            slip1=0.8;
        else
            slip1=slip_little;
        end
        if slip_big==0
            slip2=1.25;
        else
            slip2=slip_big;
        end
        if slipp==0
            slippp=0.21;
        else
            slippp=slipp;
        end
    if slip>slippp&&v_w>3; %减速，加大轮速
        y=j*v;
        i=i+1;
        j=0.99^i;
        if j<slip1
            j=slip1;
        end
    elseif slip<-slippp&&v_w>2%加速，缓加速
        y=j*v;
        i=i+1;
        j=1.01^i;
        if j>slip2
            j=slip2;
        end
    else
        y=v_e;
        i=1;
    end
    
    else
        y=v_e;
    end
    
    if v_e==0;
        y=0;
    end
end

== matlab function finalcode/Subsystem/Tx/TX控制器/控制器发送/189左后1/MATLAB Function8 ==
  data: model input; v_e input; v_w input; v input; y output; slipp input; slip_little input; slip_big input
function y = fcn(model, v_e, v_w, v, slipp, slip_little, slip_big)
    persistent i j
    if isempty(i)
        i=1;
        j=1;
    end
if model==0
    y=v_e;
else
    slip=(v-v_w)/v;
    y=v_e;

    if abs(v_e-v_w)>0.5
        if slip_little==0  %调试用
            slip1=0.8;
        else
            slip1=slip_little;
        end
        if slip_big==0
            slip2=1.25;
        else
            slip2=slip_big;
        end
        if slipp==0
            slippp=0.21;
        else
            slippp=slipp;
        end
    if slip>slippp&&v_w>3; %减速，加大轮速
        y=j*v;
        i=i+1;
        j=0.99^i;
        if j<slip1
            j=slip1;
        end
    elseif slip<-slippp&&v_w>2%加速，缓加速
        y=j*v;
        i=i+1;
        j=1.01^i;
        if j>slip2
            j=slip2;
        end
    else
        y=v_e;
        i=1;
    end
    
    else
        y=v_e;
    end
    
    if v_e==0;
        y=0;
    end
end

== matlab function finalcode/Subsystem/Tx/TX控制器/速度/184左前/MATLAB Function1 ==
  data: v input; T output; a input
function T = fcn(v,a)
% if a>5
%     y = u;
% elseif a>3&&a<5
%     y=1200;
% else
%     y=800;
% end

if v<6000*1.88e-3
    T=2100;
elseif v>11000*1.88e-3
    T=800;
else
    T=1100;
end

== matlab function finalcode/Subsystem/Tx/TX控制器/速度/188右后/MATLAB Function1 ==
  data: v input; T output; a input
function T = fcn(v,a)
% if a>5
%     y = u;
% elseif a>3&&a<5
%     y=1200;
% else
%     y=800;
% end

if v<6000*1.88e-3
    T=2100;
elseif v>11000*1.88e-3
    T=800;
else
    T=1100;
end

== matlab function finalcode/Subsystem/Rx/转向电机/Subsystem3/Subsystem/MATLAB Function ==
  data: u input; y output
function y = fcn(u)
y =   0.0003056 *u-208.4  ;
if u==683198
    y=0;
end

== matlab function finalcode/Subsystem/Tx/TX控制器/控制器发送/188右后1/MATLAB Function8 ==
  data: model input; v_e input; v_w input; v input; y output; slipp input; slip_little input; slip_big input
function y = fcn(model, v_e, v_w, v, slipp, slip_little, slip_big)
    persistent i j
    if isempty(i)
        i=1;
        j=1;
    end
if model==0
    y=v_e;
else
    slip=(v-v_w)/v;
    y=v_e;

    if abs(v_e-v_w)>0.5
        if slip_little==0  %调试用
            slip1=0.8;
        else
            slip1=slip_little;
        end
        if slip_big==0
            slip2=1.25;
        else
            slip2=slip_big;
        end
        if slipp==0
            slippp=0.21;
        else
            slippp=slipp;
        end
    if slip>slippp&&v_w>3; %减速，加大轮速
        y=j*v;
        i=i+1;
        j=0.99^i;
        if j<slip1
            j=slip1;
        end
    elseif slip<-slippp&&v_w>2%加速，缓加速
        y=j*v;
        i=i+1;
        j=1.01^i;
        if j>slip2
            j=slip2;
        end
    else
        y=v_e;
        i=1;
    end
    
    else
        y=v_e;
    end
    
    if v_e==0;
        y=0;
    end
end

== matlab function finalcode/Subsystem/run/kalman_filter1 ==
  data: a_k_1 input; y output; v_k_1 input; v_k input; V_MIN input; model input
function y = fcn(a_k_1,v_k_1,v_k,V_MIN, model)

    Z=v_k;%观测值
    %dt=0.02 ;%采样时间sampletime
    persistent X P F Q H R;%使函数退出后的计算值保持不变
    if isempty(X)% 检查是否是第一次运行，进行初始化
        X=0;%初始状态
        P=1;%状态协方差矩阵
        F=1;%状态转移矩阵
        Q=0.001;%状态转移协方差矩阵 
        H=1;%观测矩阵
        R=0.01;%观测噪声方差 

    end

    X_=v_k_1+0.01*a_k_1; %状态预测方程
    P_=F*P*F'+Q;%不确定性在各时刻的传递
    K=P_*H'/(H*P_*H'+R);%卡尔曼系数
    X=X_+K*(Z-H*X_);%状态更新
    P=(1-K*H)*P_;%噪声协方差矩阵更新
    
y=X;

if v_k<0.1||model==0||model==9||model==10
    y=V_MIN;  %即转轮时不使用惯导信息
elseif abs(X-v_k)>0.5
    y=v_k;
else
    y = X;
end
end

== matlab function finalcode/Subsystem/run/LQR ==
  data: x input; y output
function y = fcn(x)
% A=[1 1;1 1];
% size(A,1);
% B=[1;1];
% P=size(B,2);
% ts=0.02;%离散时间的步长
% sys_d=c2d(ss(A,B),ts);%连续转离散系统函数，用于仿真代码
% x0=[1,1];%系统初始化
% x=x0;
% u0=0;
% u=u0;
% Q=[1 0 ;0 1];%系统权重
% S=[1 0;0 1];%终值权重
% R=0.1;%输入权重
% %定义系统运行步数
% k_steps = 100;
% %定义x._history雩矩阵,用于储存系统状态结果
% xhistory = zeros(n ,k_steps) ;
% %俘系统状态初始值赋值到x_history矩阵第一个位置
% xhistory (:,l)= x;
% %定义u_history需矩阵,用于储存系统输入结果,
% u_history = zeros(p,k_steps) ;
% %俘系统输入初始值赋值到u_history矩阵第一个位置
% u_history (:,1) = u;
% P_k = s;
% %计算最优反馈增益
% 
% 
% % 计算最优反馈增益
% for k = l : N
% % 计算F[N-k]
% F= inv(R+B'*P_k*B)*B'*P_k*A;
% 
% N= k_steps;
% P_k = s;
% % 计算最优反馈增益
% 
% P_k = (A-B*F)'*P_k*(A-B*F)+(F)'*R*(F)+Q;
% if k ==l
% F_N=F;
% else
% F_N=[F;F_N];
% end
% %仿真开始,建立for循环
% for k=l:k_steps
% u =-FN((k-1)*p+l:k*p ,:)*x;
% x= A*x+B*u ;
% %保存系统状态到预先定义矩阵的相应位置
% x_history(: ,k+l)=x;
% %保存系统输入到预先定义矩阵的相应位置
% u_history ( :,k)=u ;
% end
% 
% y=u;

== matlab function finalcode/Subsystem/run/MATLAB Function ==
  data: NT input; u input; y output; u1 input; model input
function y = fcn(NT, u,u1,model)
if ((u>0.8&&(model==0||model==10))||(u1>0.8))||(NT<-100)
    y = 1;
else
    y=0;
end

== matlab function finalcode/Subsystem/run/MATLAB Function1 ==
  data: V_lon input; V_longitudinal output; V_lat input; theta_deg input; V_lateral output; V_MIN input
function [V_longitudinal, V_lateral] = calculateVelocities(V_lon, V_lat, theta_deg,V_MIN)
    % 将角度转换为弧度
    theta_rad = deg2rad(theta_deg);

    % 计算纵向速度和横向速度
    V_longitudinal_ = V_lon * sin(theta_rad) + V_lat * cos(theta_rad);
    if V_longitudinal_<0.2
         V_longitudinal=V_MIN;
    else
         V_longitudinal= V_longitudinal_;
    end
    V_lateral = V_lon * cos(theta_rad) -V_lat * sin(theta_rad);
end

== matlab function finalcode/Subsystem/Tx/TX控制器/速度/184左前/MATLAB Function5 ==
  data: v input; y output; angle input; vz input; model input
function y = fcn(v, angle, vz,model)
if(angle>3||angle<-3)&&model==3%4650000,4870000,4741002
    y=vz*594.06;
else
    y = v;
end

== matlab function finalcode/Subsystem/run/MATLAB Function2 ==
  data: u input; y output
function y = fcn(u)
if u>500
    y=1;
elseif u>1500
    y=2;
else
    y=0;
end

== matlab function finalcode/Subsystem/run/analog_input/MATLAB Function ==
  data: u input; y output
function y = fcn(u)
if u==9
    y=1;
else
    y=0;
end

== matlab function finalcode/Subsystem/run/analog_input/MATLAB Function1 ==
  data: u input; y output; a input
function y = fcn(u,a)
if u==1
    y=15;%%无人规则缓慢转轮
else
    y=a;
end
end

== matlab function finalcode/Subsystem/run/analog_input/MATLAB Function2 ==
  data: u input; y output; canok input
function y = fcn(u,canok)
if u==0%&&canok==1
    y=1;
else
    y=0;
end

== matlab function finalcode/Subsystem/run/analog_input/MATLAB Function3 ==
  data: model input; y output; workstation input; v input
function y = fcn(model,workstation,v)
if model~=0&&model~=10
    y=1;
else
    y=0;
end
% if canok==0
%     y=0;
% end
%  if workstation<=0.1
%      y=0;
%  end
%  if v<0.5||v>18
%      y=0;
%  end

== matlab function finalcode/Subsystem/Tx/TX控制器/速度/189左后/MATLAB Function1 ==
  data: v input; T output; a input
function T = fcn(v,a)
% if a>5
%     y = u;
% elseif a>3&&a<5
%     y=1200;
% else
%     y=800;
% end

if v<6000*1.88e-3
    T=2100;
elseif v>11000*1.88e-3
    T=800;
else
    T=1100;
end

== matlab function finalcode/Subsystem/Tx/esc，ABS/MATLAB Function ==
  data: u input; y output
function y = fcn(u)
if u~=0&&u~=9&&u~=2
    y=1;
else
    y=0;
end

== matlab function finalcode/Subsystem/run/analog_input/MATLAB Function4 ==
  data: u input; y output; a input
function y = fcn(u,a)
if u==5
    y=0;
else
    y=a;
end
end

== matlab function finalcode/Subsystem/Rx/工作站/Subsystem3/Subsystem/MATLAB Function ==
  data: u input; y output; CANOK_20 input
function y = fcn(u,CANOK_20)
if CANOK_20==0
    y=0;
else
    y=u;
end

== matlab function finalcode/Subsystem/run/analog_input/MATLAB Function5 ==
  data: u input; y output; model input; y6 output
function [y,y6] = fcn(u,model)
if model==8
    y = 0;
    y6=u;
else
    y=u;
    y6=0;
end
if y~=0&&y6~=0
    y=0;
    y6=0;
end
    
end

== matlab function finalcode/Subsystem/Rx/工作站/Subsystem3/Subsystem/MATLAB Function1 ==
  data: u input; y output; CANOK_20 input
function y = fcn(u,CANOK_20)
% if CANOK_20==0
%     y=0;
% else
    y=u;
% end

== matlab function finalcode/Subsystem/Tx/转向/MATLAB Function1 ==
  data: model input; y output; status input
function y = fcn(model,status)
if (model==1||model==3||model==4||model==5||model==6||model==7||model==8)&&(status==3||status==4||status==5||status==6)
    y=1;
else
    y=0;
end

if model==8||model==9
    y=1;
else
    y=y;
end

== matlab function finalcode/Subsystem/Tx/TX控制器/速度/184左前/MATLAB Function6 ==
  data: v input; T output; a input
function T = fcn(v,a)
% if a>5
%     y = u;
% elseif a>3&&a<5
%     y=1200;
% else
%     y=800;
% end

if v<6000*1.88e-3
    T=2100;
elseif v>11000*1.88e-3
    T=800;
else
    T=1100;
end

== matlab function finalcode/Subsystem/Tx/转向/转向换算/MATLAB Function ==
  data: biaozhi1 output; baocuo input; statu input; diaoxian input
function biaozhi1  = fcn(baocuo, statu, diaoxian)
persistent i;
     % 初始化状态变量
    if isempty(i)
        i = 1;
    end
    if baocuo==1||(statu==4&&diaoxian==0)
        i=1;
    end
    if i>4
        biaozhi1=1;
    else
        biaozhi1=0;       
    end
i=i+1;
end

== matlab function finalcode/Subsystem/Tx/转向/转向换算/Subsystem/MATLAB Function ==
  data: steer output; y output; x input; canok input; baocuo input; k input; d input; rm input; lm input
function [steer,y] = fcn(x,canok,baocuo,k,d,rm,lm)
  persistent i previoussteer;
     % 初始化状态变量
     rm=rm-3000;
     lm=lm+3000;
    if isempty(i)
        i = 0;
    end
    if isempty(previoussteer)
        previoussteer= d;
    end
    if i>0.2     
        steer= k *x+d ;
%         if x==0
%             steer=25092;
%         end
          if steer>rm
              steer=rm;
          end
          if steer<lm
              steer=lm;
          end
    else
        steer=d;
    end
    if canok==0
        steer=previoussteer;
    end
    if baocuo==1
        steer=previoussteer;
    end
    i=i+0.02;
  persistent time  a b;
     % 初始化状态变量
    if isempty(time) 
        time = 0;
   
        a=5;
        b=10;
    end
    if baocuo==1
        time=-4;
    end
    if mod(abs(time), 2) == 0
        result = 1;
    else
        result = 0;
    end
    if time<b&&result==0
    y=6;
 
    elseif time<b&&result==1
    y=15;
  
    elseif time>=b
        if result==1
            y=79;
        else
            y=63;
        end
    else
        y=6;
    end   
    time=time+1;
    previoussteer=steer;
%     
%       persistent time1;
%      % 初始化状态变量
%     if isempty(time1)
%         time1 = 0;
%     end
%     if mod(time1, 2) == 0
%         result1 = 1;
%     else
%         result1 = 0;
%     end
%     if time1<2
%     y=6;
%  
%     elseif time1>=2&&time1<4
%     y=15;
%   
%     elseif time1>=4
%         if result1==1
%             y=79;
%         else
%             y=63;
%         end
%     else
%         y=6;
%     end   
%     time1=time1+1;
   
end

== matlab function finalcode/Subsystem/Rx/工作站/Subsystem3/Subsystem/MATLAB Function2 ==
  data: u input; y output; CANOK_20 input
function y = fcn(u, CANOK_20)
    if u==0
        y=0;
    else
        y=u/100;
    end
    
    if CANOK_20==0
    y=0;
    end
end

== matlab function finalcode/Subsystem/Rx/283 285左前/Subsystem2/Subsystem/MATLAB Function ==
  data: u input; y output
function y = fcn(u)

y = u/594.06;

== matlab function finalcode/Subsystem/Rx/284 286右前/Subsystem2/Subsystem/MATLAB Function ==
  data: u input; y output
function y = fcn(u)


y = u/594.06;

== matlab function finalcode/Subsystem/Rx/288 290左后/Subsystem2/Subsystem/MATLAB Function ==
  data: u input; y output
function y = fcn(u)


y = u/594.06;
